simulink model "uz_mpc_cost_and_optim_state_machine"  (R2021a)
settings: Solver=FixedStepAuto  StartTime=0.0  StopTime=10000*t_ADC  RelTol=1e-3
values from neighbouring files (symbols this model uses):
  A = 1.0    (= 1)    [uz_6ph_pu_vsd_voltages_init.m]    (also in uz_mpc_6ph_init.m; uz_mpc_6ph_state_machine_init.m = 0.1)
  f = n_rpm/60.0*p    (= 250)    [uz_6ph_pu_vsd_voltages_init.m]    (also in uz_mpc_6ph_init.m; uz_mpc_6ph_state_machine_init.m = 83.3333333333)
  IB = sqrt(2)*IR    [uz_6ph_pu_vsd_voltages_init.m]    (also in uz_mpc_6ph_init.m; uz_mpc_6ph_state_machine_init.m)
  id_ref = 0.0    (= 0)    [uz_6ph_pu_vsd_voltages_init.m]    (also in uz_mpc_6ph_init.m; uz_mpc_6ph_state_machine_init.m)
  iq_ref = -10.0    (= -10)    [uz_6ph_pu_vsd_voltages_init.m]    (also in uz_mpc_6ph_init.m; uz_mpc_6ph_state_machine_init.m = 5)
  ix_ref = 0.0    (= 0)    [uz_6ph_pu_vsd_voltages_init.m]    (also in uz_mpc_6ph_init.m; uz_mpc_6ph_state_machine_init.m)
  iy_ref = 0.0    (= 0)    [uz_6ph_pu_vsd_voltages_init.m]    (also in uz_mpc_6ph_init.m; uz_mpc_6ph_state_machine_init.m)
  lambda_d = 1.0    (= 1)    [uz_mpc_6ph_state_machine_init.m]
  lambda_q = 1.0    (= 1)    [uz_mpc_6ph_state_machine_init.m]
  lambda_u = 0.0    (= 0)    [uz_mpc_6ph_state_machine_init.m]
  lambda_x = 0.1    [uz_mpc_6ph_state_machine_init.m]
  lambda_y = 0.1    [uz_mpc_6ph_state_machine_init.m]
  Ld_over_LB = Ld/LB    [uz_6ph_pu_vsd_voltages_init.m]    (also in uz_mpc_6ph_init.m; uz_mpc_6ph_state_machine_init.m)
  Lq_over_LB = Lq/LB    [uz_6ph_pu_vsd_voltages_init.m]    (also in uz_mpc_6ph_init.m; uz_mpc_6ph_state_machine_init.m)
  n_rpm = 3000    [uz_6ph_pu_vsd_voltages_init.m]    (also in uz_mpc_6ph_init.m; uz_mpc_6ph_state_machine_init.m = 1000)
  omega_m = n_rpm*pi/30    (= 314.159265359)    [uz_6ph_pu_vsd_voltages_init.m]    (also in uz_mpc_6ph_init.m; uz_mpc_6ph_state_machine_init.m = 104.71975512)
  omegaB = nR*2*pi()/60*p    [uz_6ph_pu_vsd_voltages_init.m]    (also in uz_mpc_6ph_init.m; uz_mpc_6ph_state_machine_init.m)
  p = 5    [uz_6ph_pu_vsd_voltages_init.m]    (also in uz_mpc_6ph_init.m; uz_mpc_6ph_state_machine_init.m)
  psi_pm_over_psiB = psi_pm/psiB    [uz_6ph_pu_vsd_voltages_init.m]    (also in uz_mpc_6ph_init.m; uz_mpc_6ph_state_machine_init.m)
  Rs_over_ZB = Rs/ZB    [uz_6ph_pu_vsd_voltages_init.m]    (also in uz_mpc_6ph_init.m; uz_mpc_6ph_state_machine_init.m)
  t_ADC = 1/f_ADC    (= 1e-05)    [uz_6ph_pu_vsd_voltages_init.m]    (also in uz_mpc_6ph_init.m; uz_mpc_6ph_state_machine_init.m; uz_typeconv_init.m)
  t_clock = 1/f_clock    (= 1e-08)    [uz_6ph_pu_vsd_voltages_init.m]    (also in uz_mpc_6ph_init.m; uz_mpc_6ph_state_machine_init.m; uz_typeconv_init.m)
  Ts_times_ZB_over_Ld = Ts*ZB/Ld    [uz_6ph_pu_vsd_voltages_init.m]    (also in uz_mpc_6ph_init.m; uz_mpc_6ph_state_machine_init.m)
  Ts_times_ZB_over_Lq = Ts*ZB/Lq    [uz_6ph_pu_vsd_voltages_init.m]    (also in uz_mpc_6ph_init.m; uz_mpc_6ph_state_machine_init.m)
  Ts_times_ZB_over_Lx = Ts*ZB/Lx    [uz_6ph_pu_vsd_voltages_init.m]    (also in uz_mpc_6ph_init.m; uz_mpc_6ph_state_machine_init.m)
  Ts_times_ZB_over_Ly = Ts*ZB/Ly    [uz_6ph_pu_vsd_voltages_init.m]    (also in uz_mpc_6ph_init.m; uz_mpc_6ph_state_machine_init.m)
  v_dc = 565.0    (= 565)    [uz_6ph_pu_vsd_voltages_init.m]    (also in uz_mpc_6ph_init.m; uz_mpc_6ph_state_machine_init.m)
  VB = sqrt(2/3)*VR    [uz_6ph_pu_vsd_voltages_init.m]    (also in uz_mpc_6ph_init.m; uz_mpc_6ph_state_machine_init.m)
libraries: nesl_utility x38, fl_lib x30, ee_lib x14, simulink x10, hdlsllib x2
(part 2 of 3)

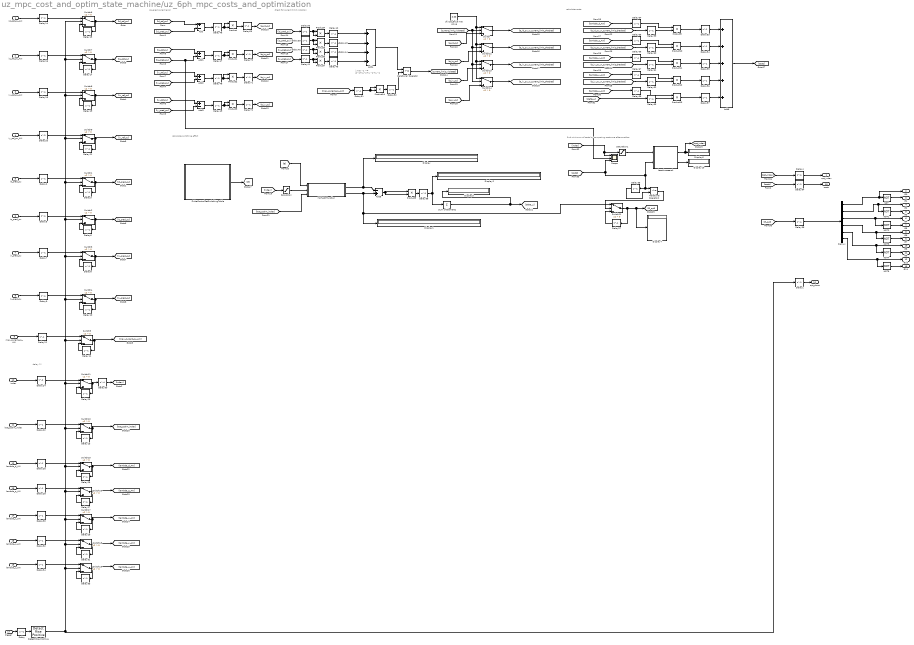
== system uz_mpc_cost_and_optim_state_machine/uz_6ph_mpc_costs_and_optimization ==
  note: delay 2 !
  note: i_max^2 <= id^2+iq^2+ix^2+iy^2
  note: find minimum of costs by comparing costs one after another
  note: calculate costs
  note: calculate switching effort
  note: check for current limit violation
  note: squared current error
  id_ref_pu_AXI : Inport
  iq_ref_pu_AXI : Inport  Port=2
  ix_ref_pu_AXI : Inport  Port=3
  iy_ref_pu_AXI : Inport  Port=4
  id_pred_pu : Inport  Port=5
  iq_pred_pu : Inport  Port=6
  ix_pred_pu : Inport  Port=7
  iy_pred_pu : Inport  Port=8
  max_current_pu_AXI : Inport  Port=9
  index : Inport  Port=10
  last_optim_index : Inport  Port=11
  lambda_d_AXI : Inport  Port=12
  lambda_q_AXI : Inport  Port=13
  lambda_x_AXI : Inport  Port=14
  lambda_y_AXI : Inport  Port=15
  lambda_u_AXI : Inport  Port=16
  trigger : Inport  Port=17
  Add{,1..3} (4 alike) : Sum  Inputs=+-
  Add4 : Sum  Inputs=++++  AccumDataTypeStr=fixdt_type_squared_current_error
  Add5 : Sum  Inputs=-+
  Add6 : Sum  Inputs=+++++  AccumDataTypeStr=fixdt_type_delta_u_costs
  Delay{,1..12,14..21,25..34,36,38..49,51..72,94} (67 alike) : Delay  DelayLength=1
  Delay13 : Delay  DelayLength=1  InitialCondition=1
  Delay22 : Delay  DelayLength=1  InitialCondition=1
  Delay23 : Delay  DelayLength=1  InitialCondition=1
  Delay24 : Delay  InitialCondition=1
  Delay35 : Delay  DelayLength=1  InitialCondition=4.99
  Delay37 : Delay  DelayLength=1  InitialCondition=0
  Delay50 : Delay  DelayLength=4  InitialCondition=1
  Demux : Demux  Outputs=6
  Detect Rise Positive : simulink/Logic and Bit Operations/Detect Rise Positive  vinit=0  OutDataTypeStr=boolean
  Display{,1..3,6..7,10} (7 alike) : Display
  FiniteControlSetSwitchingTable : MATLAB Function  TreatAsAtomicUnit=on
  MATLAB Function : MATLAB Function  TreatAsAtomicUnit=on
  NOT{,1..5} (6 alike) : Logic  Operator=NOT  IconShape=distinctive  AllPortsSameDT=off  OutDataTypeStr=boolean
  Product{,1..7,9..12,14} (13 alike) : Product  OutDataTypeStr=fixdt_type_squared_current_error
  Product13 : Product  OutDataTypeStr=fixdt_type_delta_u_costs
  Product8 : Product  OutDataTypeStr=uint16
  Relational Operator : RelationalOperator  OutDataTypeStr=boolean  RndMeth=Simplest
  Relational Operator1 : RelationalOperator  Operator=<=  OutDataTypeStr=boolean  RndMeth=Simplest
  Saturation : Saturate  UpperLimit=64  LowerLimit=1
  Saturation1 : Saturate  UpperLimit=64  LowerLimit=1
  Scope : Scope  NumInputPorts=3
  Sum of Elements : Sum  Inputs=+  AccumDataTypeStr=uint16
  Switch{,1..19,21} (21 alike) : Switch  Criteria=u2 > Threshold
  iterativesearch : MATLAB Function  TreatAsAtomicUnit=on
  sfix18_En15 max value : Constant  Value=3.99  OutDataTypeStr=fixdt(1,18,15)  SampleTime=-1
  opt_index : Outport  VectorParamsAs1DForOutWhenUnconnected=off
  G0 : Outport  Port=2  VectorParamsAs1DForOutWhenUnconnected=off
  G1 : Outport  Port=3  VectorParamsAs1DForOutWhenUnconnected=off
  G2 : Outport  Port=4  VectorParamsAs1DForOutWhenUnconnected=off
  G3 : Outport  Port=5  VectorParamsAs1DForOutWhenUnconnected=off
  G4 : Outport  Port=6  VectorParamsAs1DForOutWhenUnconnected=off
  G5 : Outport  Port=7  VectorParamsAs1DForOutWhenUnconnected=off
  G6 : Outport  Port=8  VectorParamsAs1DForOutWhenUnconnected=off
  G7 : Outport  Port=9  VectorParamsAs1DForOutWhenUnconnected=off
  G8 : Outport  Port=10  VectorParamsAs1DForOutWhenUnconnected=off
  G9 : Outport  Port=11  VectorParamsAs1DForOutWhenUnconnected=off
  G10 : Outport  Port=12  VectorParamsAs1DForOutWhenUnconnected=off
  G11 : Outport  Port=13  VectorParamsAs1DForOutWhenUnconnected=off
  opt_done : Outport  Port=14  VectorParamsAs1DForOutWhenUnconnected=off
  costs : Outport  Port=15  VectorParamsAs1DForOutWhenUnconnected=off
  wires:
  trigger/1 -> Delay/1
  Delay/1 -> Detect Rise Positive/1
  Delay1/1 -> opt_done/1
  Delay4/1 -> opt_index/1
  Switch9/1 -> [iy_ref_pu], Delay21/1
  Delay17/1 -> Switch7/3
  id_ref_pu_AXI/1 -> Delay14/1
  Delay18/1 -> Switch8/1
  Switch8/1 -> [ix_ref_pu], Delay19/1
  Delay21/1 -> Switch9/3
  Switch7/1 -> [iq_ref_pu], Delay17/1
  iy_ref_pu_AXI/1 -> Delay20/1
  iq_ref_pu_AXI/1 -> Delay16/1
  Delay16/1 -> Switch7/1
  Delay19/1 -> Switch8/3
  Delay20/1 -> Switch9/1
  Delay15/1 -> Switch6/3
  Switch6/1 -> [id_ref_pu], Delay15/1
  ix_ref_pu_AXI/1 -> Delay18/1
  Delay14/1 -> Switch6/1
  Switch1/1 -> [id_pred_pu], Delay3/1
  ix_pred_pu/1 -> Delay7/1
  Delay9/1 -> Switch4/1
  Delay2/1 -> Switch1/1
  Delay8/1 -> Switch3/3
  Delay5/1 -> Switch2/1
  iy_pred_pu/1 -> Delay9/1
  iq_pred_pu/1 -> Delay5/1
  Switch3/1 -> Delay8/1, [ix_pred_pu]
  Delay10/1 -> Switch4/3
  Switch2/1 -> [iq_pred_pu], Delay6/1
  Delay7/1 -> Switch3/1
  Switch4/1 -> [iy_pred_pu], Delay10/1
  Delay6/1 -> Switch2/3
  Delay3/1 -> Switch1/3
  id_pred_pu/1 -> Delay2/1
  max_current_pu_AXI/1 -> Delay12/1
  Delay12/1 -> Switch5/1
  Delay11/1 -> Switch5/3
  Switch5/1 -> [max_current_pu_AXI], Delay11/1
  last_optim_index/1 -> Delay22/1
  Delay22/1 -> Switch10/1
  Delay13/1 -> Switch10/3
  Switch10/1 -> [last_optim_index], Delay13/1
  FiniteControlSetSwitchingTable/1(G) -> [G]
  Delay24/1 -> Switch11/1
  index/1 -> Delay24/1
  Delay23/1 -> Switch11/3
  Switch11/1 -> Delay50/1, Delay23/1
  [e_id_pu] -> Switch/3
  [current_limit_violated] -> Switch13/2, Switch14/2, Switch12/2, Switch/2
  [e_iq_pu] -> Switch12/3
  [e_ix_pu] -> Switch13/3
  sfix18_En15 max value/1 -> Switch/1, Switch14/1, Switch13/1, Switch12/1
  [e_iy_pu] -> Switch14/3
  [G] -> MATLAB Function/1(in)
  Delay26/1 -> Switch15/1
  Delay25/1 -> Switch15/3
  Switch15/1 -> [lambda_d_AXI], Delay25/1
  lambda_d_AXI/1 -> Delay26/1
  lambda_q_AXI/1 -> Delay28/1
  Delay28/1 -> Switch16/1
  Switch16/1 -> [lambda_q_AXI], Delay27/1
  Delay27/1 -> Switch16/3
  lambda_y_AXI/1 -> Delay32/1
  Switch18/1 -> [lambda_y_AXI], Delay31/1
  Delay31/1 -> Switch18/3
  Delay32/1 -> Switch18/1
  lambda_x_AXI/1 -> Delay30/1
  Delay30/1 -> Switch17/1
  Switch17/1 -> [lambda_x_AXI], Delay29/1
  Delay29/1 -> Switch17/3
  Delay33/1 -> Switch19/3
  Switch19/1 -> [lambda_u_AXI], Delay33/1
  lambda_u_AXI/1 -> Delay34/1
  Delay34/1 -> Switch19/1
  [opt_index] -> Delay4/1
  Delay38/1 -> Demux/1
  Add4/1 -> Relational Operator/1
  NOT/1 -> G1/1
  Demux/1 -> G0/1, NOT/1
  NOT5/1 -> G11/1
  NOT4/1 -> G9/1
  NOT3/1 -> G7/1
  NOT2/1 -> G5/1
  NOT1/1 -> G3/1
  Demux/2 -> NOT1/1, G2/1
  Demux/3 -> NOT2/1, G4/1
  Demux/4 -> NOT3/1, G6/1
  Demux/5 -> NOT4/1, G8/1
  Demux/6 -> NOT5/1, G10/1
  Product8/1 -> Delay58/1
  Sum of Elements/1 -> [delta_u], Display3/1
  Add5/1 -> Product8/1, Product8/2
  MATLAB Function/1(G_next) -> Display/1, Add5/1
  Product9/1 -> Delay53/1
  Product10/1 -> Delay54/1
  Product11/1 -> Delay55/1
  Product12/1 -> Delay56/1
  Product13/1 -> Delay57/1
  Add6/1 -> [costs]
  [lambda_d_AXI] -> Delay64/1
  [lambda_q_AXI] -> Delay65/1
  [lambda_x_AXI] -> Delay66/1
  [lambda_y_AXI] -> Delay67/1
  [lambda_u_AXI] -> Delay68/1
  [delta_u] -> Delay63/1
  [e_id_pu_w_current_limit_checked] -> Delay59/1
  [e_iy_pu_w_current_limit_checked] -> Delay62/1
  [e_ix_pu_w_current_limit_checked] -> Delay61/1
  [e_iq_pu_w_current_limit_checked] -> Delay60/1
  [id_ref_pu] -> Add/1
  [id_pred_pu] -> Add/2
  [iq_pred_pu] -> Scope/2, Add1/2
  [iq_ref_pu] -> Add1/1
  [ix_ref_pu] -> Add2/1
  [ix_pred_pu] -> Add2/2
  [iy_ref_pu] -> Add3/1
  [iy_pred_pu] -> Add3/2
  Add3/1 -> Delay49/1
  Add1/1 -> Delay47/1
  Add2/1 -> Delay48/1
  Add/1 -> Delay46/1
  Product3/1 -> Delay72/1
  Product2/1 -> Delay71/1
  Product1/1 -> Delay70/1
  Product/1 -> Delay69/1
  Product4/1 -> Delay42/1
  Product5/1 -> Delay43/1
  Product6/1 -> Delay44/1
  Product7/1 -> Delay45/1
  [id_pred_pu] -> Delay36/1
  [iq_pred_pu] -> Delay39/1
  [ix_pred_pu] -> Delay40/1
  [iy_pred_pu] -> Delay41/1
  Relational Operator/1 -> [current_limit_violated]
  Switch14/1 -> [e_iy_pu_w_current_limit_checked]
  Switch13/1 -> [e_ix_pu_w_current_limit_checked]
  Switch12/1 -> [e_iq_pu_w_current_limit_checked]
  Switch/1 -> [e_id_pu_w_current_limit_checked]
  [max_current_pu_AXI] -> Delay51/1
  Product14/1 -> Delay52/1
  [costs] -> Delay94/1
  Delay94/1 -> costs/1
  Delay37/1 -> Switch21/3
  Switch21/1 -> Display7/1, [G_opt], Delay37/1
  Detect Rise Positive/1 -> Switch4/2, Switch3/2, Switch2/2, Switch1/2, Switch6/2, Switch7/2, Switch8/2, Switch9/2, Switch5/2, Switch11/2, Switch10/2, Switch15/2, Switch16/2, Switch17/2, Switch18/2, Switch19/2, Delay1/1
  MATLAB Function/2(G_prev) -> Add5/2, Display1/1, Switch21/1
  [last_optim_index] -> MATLAB Function/3(last_optim_index)
  [costs] -> Scope/3, Delay35/1, Relational Operator1/1, iterativesearch/2(cost)
  [index] -> Scope/1, Saturation1/1
  [index] -> Saturation/1
  Saturation/1 -> MATLAB Function/2(index)
  Saturation1/1 -> iterativesearch/1(index)
  Delay35/1 -> Relational Operator1/2
  Relational Operator1/1 -> Switch21/2
  [G_opt] -> Delay38/1
  iterativesearch/1(opt_idx) -> [opt_index], Display6/1
  iterativesearch/2(min_costs) -> Display10/1
  Delay36/1 -> Product4/2, Product4/1
  Delay39/1 -> Product5/2, Product5/1
  Delay40/1 -> Product6/2, Product6/1
  Delay41/1 -> Product7/2, Product7/1
  Delay44/1 -> Add4/3
  Delay42/1 -> Add4/1
  Delay45/1 -> Add4/4
  Delay43/1 -> Add4/2
  Delay46/1 -> Product/1, Product/2
  Delay47/1 -> Product1/1, Product1/2
  Delay48/1 -> Product2/1, Product2/2
  Delay49/1 -> Product3/1, Product3/2
  Delay50/1 -> [index]
  Delay51/1 -> Product14/1, Product14/2
  Delay52/1 -> Relational Operator/2
  Delay53/1 -> Add6/1
  Delay54/1 -> Add6/2
  Delay55/1 -> Add6/3
  Delay56/1 -> Add6/4
  Delay57/1 -> Add6/5
  Delay58/1 -> Sum of Elements/1, Display2/1
  Delay59/1 -> Product9/2
  Delay60/1 -> Product10/2
  Delay61/1 -> Product11/2
  Delay62/1 -> Product12/2
  Delay63/1 -> Product13/2
  Delay64/1 -> Product9/1
  Delay65/1 -> Product10/1
  Delay66/1 -> Product11/1
  Delay67/1 -> Product12/1
  Delay68/1 -> Product13/1
  Delay69/1 -> [e_id_pu]
  Delay70/1 -> [e_iq_pu]
  Delay71/1 -> [e_ix_pu]
  Delay72/1 -> [e_iy_pu]

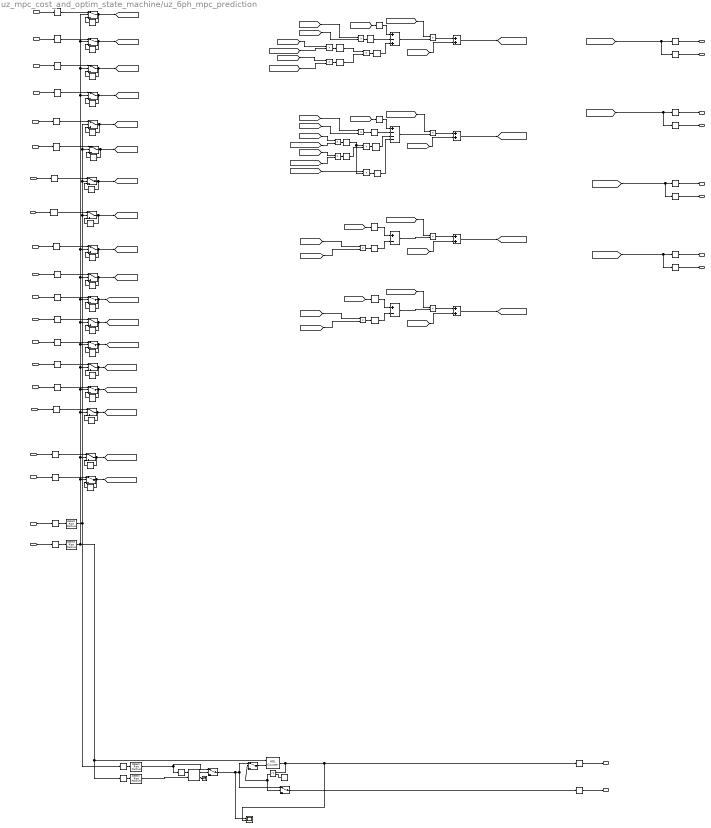
== system uz_mpc_cost_and_optim_state_machine/uz_6ph_mpc_prediction ==
  note: voltages are triggered from voltage calculation ip every iteration
  note: iy_delay_pu = Ts_times_ZB_over_Ly *(vy_pu - Rs_over_ZB * iy_k_pu) + iy_k_pu
  note: ix_delay_pu = Ts_times_ZB_over_Lx *(vx_pu - Rs_over_ZB* ix_k_pu) + ix_k_pu
  note: iq_delay_pu = Ts_times_ZB_over_Lq *(vq_pu - Rs_over_ZB * iq_k_pu - omega_m_pu * polepairs * Ld_over_LB * id_k_pu - omega_m_pu * polepairs * psi_pm_over_psiB) + iq_k_pu
  note: id_delay_pu = Ts_times_ZB_over_Ld *(vd_pu - Rs_over_ZB * id_k_pu + iq_k_pu * Lq_over_LB * omega_m_pu * polepairs) + id_k_pu
  note: mpc state machine
  id_pu : Inport  OutDataTypeStr=fixdt_type_dq_currents
  iq_pu : Inport  Port=2  OutDataTypeStr=fixdt_type_dq_currents
  ix_pu : Inport  Port=3  OutDataTypeStr=fixdt_type_xy_currents
  iy_pu : Inport  Port=4  OutDataTypeStr=fixdt_type_xy_currents
  vd_pu : Inport  Port=5  OutDataTypeStr=fixdt_type_dqxy_voltages
  vq_pu : Inport  Port=6  OutDataTypeStr=fixdt_type_dqxy_voltages
  vx_pu : Inport  Port=7  OutDataTypeStr=fixdt_type_dqxy_voltages
  vy_pu : Inport  Port=8  OutDataTypeStr=fixdt_type_dqxy_voltages
  omega_m_pu : Inport  Port=9  OutDataTypeStr=fixdt_type_speed
  Rs_over_ZB_AXI : Inport  Port=10  OutDataTypeStr=fixdt_type_constants
  Ts_times_ZB_over_Ld_AXI : Inport  Port=11  OutDataTypeStr=fixdt_type_constants
  Ts_times_ZB_over_Lq_AXI : Inport  Port=12  OutDataTypeStr=fixdt_type_constants
  Ts_times_ZB_over_Lx_AXI : Inport  Port=13  OutDataTypeStr=fixdt_type_constants
  Ts_times_ZB_over_Ly_AXI : Inport  Port=14  OutDataTypeStr=fixdt_type_constants
  Ld_over_LB_AXI : Inport  Port=15  OutDataTypeStr=fixdt_type_constants
  Lq_over_LB_AXI : Inport  Port=16  OutDataTypeStr=fixdt_type_constants
  psi_pm_over_psiB_AXI : Inport  Port=17  OutDataTypeStr=fixdt_type_constants
  polepairs_AXI : Inport  Port=18  OutDataTypeStr=fixdt_type_polepairs
  trigger_voltages_done : Inport  Port=19
  adc_trigger : Inport  Port=20
  Add : Sum  Inputs=+-+  AccumDataTypeStr=fixdt(1,27,16)
  Add{1,3,5,7} (4 alike) : Sum  AccumDataTypeStr=fixdt(1,27,24)
  Add2 : Sum  Inputs=+---  AccumDataTypeStr=fixdt(1,27,16)
  Add4 : Sum  Inputs=+-  AccumDataTypeStr=fixdt(1,27,16)
  Add6 : Sum  Inputs=+-  AccumDataTypeStr=fixdt(1,27,16)
  Constant : Constant  Value=63  OutDataTypeStr=uint8  SampleTime=-1
  Delay{,2,4,6,8,11..12,14..17,25,27,29,31,33,35,37,39,43,50,59..60,62..65,71,73} (29 alike) : Delay
  Delay{1,3,5,7,9..10,13,18..24,26,28,30,32,34,36,38,40..42,44..48,53..55,57..58,70,72} (36 alike) : Delay  DelayLength=1
  Delay49 : Delay  DelayLength=1  InitialCondition=0
  Detect Rise Positive{,1..3} (4 alike) : simulink/Logic and Bit Operations/Detect Rise Positive  vinit=0  OutDataTypeStr=boolean
  HDL Counter : hdlsllib/Sources/HDL Counter  CountType=Free running  CountInit=0  CountStep=1  CountMax=64  CountFromType=Initial value  CountFrom=0  CountResetPort=on  CountLoadPort=off  CountEnbPort=on  CountDirPort=off  CountHitOutputPort=off  CountDataType=Unsigned  CountWordLen=8  CountFracLen=0  CountSampTime=1
  Product{,1..2,4..7,9..14} (13 alike) : Product  OutDataTypeStr=fixdt(1,18,15)
  Product3 : Product  OutDataTypeStr=fixdt(1,27,16)
  Product8 : Product  OutDataTypeStr=fixdt(1,27,16)
  Relational Operator : RelationalOperator  Operator=<=  OutDataTypeStr=boolean  RndMeth=Simplest
  Scope : Scope  NumInputPorts=2
  Subsystem : Subsystem
  Switch : Switch  Criteria=u2 > Threshold  OutDataTypeStr=fixdt_type_dq_currents
  Switch1 : Switch  Criteria=u2 > Threshold  OutDataTypeStr=fixdt_type_dq_currents
  Switch{12..19} (8 alike) : Switch  Criteria=u2 > Threshold  OutDataTypeStr=fixdt_type_constants
  Switch2 : Switch  Criteria=u2 > Threshold  OutDataTypeStr=fixdt_type_xy_currents
  Switch21 : Switch  Criteria=u2 > Threshold  OutDataTypeStr=fixdt_type_polepairs
  Switch{28..31} (4 alike) : Switch  Criteria=u2 > Threshold  OutDataTypeStr=fixdt_type_dqxy_voltages
  Switch3 : Switch  Criteria=u2 > Threshold  OutDataTypeStr=fixdt_type_xy_currents
  Switch4 : Switch  Criteria=u2 > Threshold
  Switch5 : Switch  Criteria=u2 > Threshold  OutDataTypeStr=fixdt_type_speed
  Switch6 : Switch  Criteria=u2 > Threshold
  Switch7 : Switch  Criteria=u2 > Threshold
  Terminator1 : Terminator
  id_pred_pu : Outport
  iq_pred_pu : Outport  Port=2
  ix_pred_pu : Outport  Port=3
  iy_pred_pu : Outport  Port=4
  id_pred_pu_AXI : Outport  Port=5
  iq_pred_pu_AXI : Outport  Port=6
  ix_pred_pu_AXI : Outport  Port=7
  iy_pred_pu_AXI : Outport  Port=8
  prediction_done : Outport  Port=9
  index : Outport  Port=10  VectorParamsAs1DForOutWhenUnconnected=off
  wires:
  Add5/1 -> [ix_delay_pu]
  Switch12/1 -> [Rs_over_ZB_AXI], Delay26/1
  Add3/1 -> [iq_delay_pu]
  Add1/1 -> [id_delay_pu]
  Add7/1 -> [iy_delay_pu]
  Delay5/1 -> Switch1/3
  Delay25/1 -> Switch12/1
  Delay59/1 -> Switch28/1
  Delay33/1 -> Switch16/1
  vx_pu/1 -> Delay71/1
  vd_pu/1 -> Delay59/1
  Switch15/1 -> [Ts_times_ZB_over_Lx_AXI], Delay32/1
  Ld_over_LB_AXI/1 -> Delay35/1
  Delay2/1 -> Switch/1
  Switch16/1 -> Delay34/1, [Ts_times_ZB_over_Ly_AXI]
  ix_pu/1 -> Delay6/1
  Delay38/1 -> Switch18/3
  Switch17/1 -> Delay36/1, [Ld_over_LB_AXI]
  Delay9/1 -> Switch3/3
  Switch13/1 -> [Ts_times_ZB_over_Ld_AXI], Delay28/1
  Delay/1 -> Detect Rise Positive/1
  Delay34/1 -> Switch16/3
  Delay44/1 -> Switch21/3
  Delay29/1 -> Switch14/1
  Delay8/1 -> Switch3/1
  Switch29/1 -> [vq_pu], Delay58/1
  Switch3/1 -> [iy_pu], Delay9/1
  polepairs_AXI/1 -> Delay43/1
  Delay72/1 -> Switch31/3
  Delay43/1 -> Switch21/1
  Switch14/1 -> [Ts_times_ZB_over_Lq_AXI], Delay30/1
  Delay28/1 -> Switch13/3
  psi_pm_over_psiB_AXI/1 -> Delay39/1
  Delay58/1 -> Switch29/3
  id_pu/1 -> Delay2/1
  Switch21/1 -> [polepairs_AXI], Delay44/1
  Switch/1 -> [id_pu], Delay3/1
  Delay35/1 -> Switch17/1
  Delay31/1 -> Switch15/1
  Switch28/1 -> [vd_pu], Delay57/1
  Ts_times_ZB_over_Ly_AXI/1 -> Delay33/1
  Delay7/1 -> Switch2/3
  Delay37/1 -> Switch18/1
  Delay4/1 -> Switch1/1
  Switch2/1 -> [ix_pu], Delay7/1
  Delay12/1 -> Switch5/1
  Delay73/1 -> Switch31/1
  Switch31/1 -> Delay72/1, [vy_pu]
  omega_m_pu/1 -> Delay12/1
  Delay6/1 -> Switch2/1
  Delay27/1 -> Switch13/1
  vq_pu/1 -> Delay60/1
  Switch5/1 -> [omega_m_pu], Delay13/1
  Lq_over_LB_AXI/1 -> Delay37/1
  iq_pu/1 -> Delay4/1
  iy_pu/1 -> Delay8/1
  vy_pu/1 -> Delay73/1
  Delay70/1 -> Switch30/3
  Delay60/1 -> Switch29/1
  Switch30/1 -> Delay70/1, [vx_pu]
  Ts_times_ZB_over_Lq_AXI/1 -> Delay29/1
  Delay3/1 -> Switch/3
  Switch18/1 -> Delay38/1, [Lq_over_LB_AXI]
  Delay26/1 -> Switch12/3
  Switch19/1 -> [psi_pm_over_psiB_AXI], Delay40/1
  Ts_times_ZB_over_Lx_AXI/1 -> Delay31/1
  Delay71/1 -> Switch30/1
  Switch1/1 -> [iq_pu], Delay5/1
  Ts_times_ZB_over_Ld_AXI/1 -> Delay27/1
  Delay57/1 -> Switch28/3
  Rs_over_ZB_AXI/1 -> Delay25/1
  Delay39/1 -> Switch19/1
  adc_trigger/1 -> Delay/1
  Delay40/1 -> Switch19/3
  Delay13/1 -> Switch5/3
  Delay32/1 -> Switch15/3
  Delay36/1 -> Switch17/3
  Delay30/1 -> Switch14/3
  Delay11/1 -> prediction_done/1
  [iy_delay_pu] -> Delay17/1, Delay65/1
  [iq_delay_pu] -> Delay15/1, Delay63/1
  [id_delay_pu] -> Delay14/1, Delay62/1
  Delay63/1 -> iq_pred_pu_AXI/1
  Delay65/1 -> iy_pred_pu_AXI/1
  Delay64/1 -> ix_pred_pu_AXI/1
  [ix_delay_pu] -> Delay16/1, Delay64/1
  Delay62/1 -> id_pred_pu_AXI/1
  Delay15/1 -> iq_pred_pu/1
  Delay14/1 -> id_pred_pu/1
  Delay16/1 -> ix_pred_pu/1
  Delay17/1 -> iy_pred_pu/1
  Add/1 -> Product/2
  [Ts_times_ZB_over_Ld_AXI] -> Product/1  "Ts_times_ZB_over_Ld"
  Product/1 -> Add1/1
  [id_pu] -> Add1/2  "id_k_pu"
  [Rs_over_ZB_AXI] -> Product1/1  "Rs_over_ZB"
  [id_pu] -> Product1/2  "id_k_pu"
  [iq_pu] -> Product3/1  "iq_k_pu"
  [Lq_over_LB_AXI] -> Product3/2  "Lq_over_LB"
  [omega_m_pu] -> Product4/1  "omega_m_pu"
  [polepairs_AXI] -> Product4/2  "polepairs"
  [Ts_times_ZB_over_Lq_AXI] -> Product5/1  "Ts_times_ZB_over_Lq"
  [iq_pu] -> Product6/2  "iq_k_pu"
  [Rs_over_ZB_AXI] -> Product6/1  "Rs_over_ZB"
  Add2/1 -> Product5/2
  [omega_m_pu] -> Product9/1  "omega_m_pu"
  [iq_pu] -> Add3/2  "iq_k_pu"
  [id_pu] -> Product8/1  "id_k_pu"
  [Ld_over_LB_AXI] -> Product8/2  "Ld_over_LB"
  [polepairs_AXI] -> Product9/2  "polepairs"
  Product5/1 -> Add3/1
  [psi_pm_over_psiB_AXI] -> Product10/1
  [Ts_times_ZB_over_Lx_AXI] -> Product11/1  "Ts_times_ZB_over_Lx"
  [ix_pu] -> Product12/2  "ix_k_pu"
  [Rs_over_ZB_AXI] -> Product12/1  "Rs_over_ZB"
  Add4/1 -> Product11/2
  [ix_pu] -> Add5/2  "ix_k_pu"
  Product11/1 -> Add5/1
  [Rs_over_ZB_AXI] -> Product14/1  "Rs_over_ZB"
  Add6/1 -> Product13/2
  [iy_pu] -> Add7/2  "iy_k_pu"
  [iy_pu] -> Product14/2  "iy_k_pu"
  [Ts_times_ZB_over_Ly_AXI] -> Product13/1  "Ts_times_ZB_over_Ly"
  Product13/1 -> Add7/1
  Product2/1 -> Delay1/1
  Product1/1 -> Delay10/1
  Delay10/1 -> Add/2
  Delay1/1 -> Add/3
  [vd_pu] -> Delay18/1  "vd_pu"
  Delay18/1 -> Add/1
  [vq_pu] -> Delay19/1  "vq_pu"
  Product7/1 -> Delay21/1
  Product10/1 -> Delay22/1
  Delay22/1 -> Add2/4
  Delay21/1 -> Add2/3
  Delay20/1 -> Add2/2
  Delay19/1 -> Add2/1
  Product6/1 -> Delay20/1
  [vx_pu] -> Delay23/1  "vx_pu"
  Delay23/1 -> Add4/1
  Product12/1 -> Delay24/1
  Delay24/1 -> Add4/2
  [vy_pu] -> Delay41/1  "vy_pu"
  Product14/1 -> Delay42/1
  Delay42/1 -> Add6/2
  Delay41/1 -> Add6/1
  Product4/1 -> Delay45/1
  Product3/1 -> Delay46/1
  Delay46/1 -> Product2/2
  Delay45/1 -> Product2/1
  Product9/1 -> Delay47/1
  Delay47/1 -> Product10/2, Product7/1
  Product8/1 -> Delay48/1
  Delay48/1 -> Product7/2
  Detect Rise Positive1/1 -> Delay53/1, Switch31/2, Switch30/2, Switch29/2, Switch28/2  "delay_comp done"
  trigger_voltages_done/1 -> Delay50/1
  Delay50/1 -> Detect Rise Positive1/1
  Switch7/1 -> Scope/1, Switch6/1, Switch4/1  "trigger_predict"
  Detect Rise Positive/1 -> Switch21/2, Switch19/2, Switch18/2, Switch17/2, Switch16/2, Switch15/2, Switch14/2, Switch13/2, Switch12/2, Switch5/2, Switch3/2, Switch2/2, Switch1/2, Switch/2, Delay54/1, HDL Counter/1
  Detect Rise Positive3/1 -> Subsystem/2(Reset)
  Delay54/1 -> Detect Rise Positive3/1
  Delay55/1 -> Subsystem/1(Set)
  Subsystem/2(!Q) -> Terminator1/1
  Detect Rise Positive2/1 -> Delay55/1, Switch7/1
  Subsystem/1(Q) -> Switch7/2  "Q"
  Delay53/1 -> Detect Rise Positive2/1
  HDL Counter/1 -> Relational Operator/1, Scope/2, Delay49/1
  Delay49/1 -> index/1
  Constant/1 -> Relational Operator/2
  Switch4/1 -> HDL Counter/2
  Relational Operator/1 -> Switch6/2, Switch4/2
  Switch6/1 -> Delay11/1

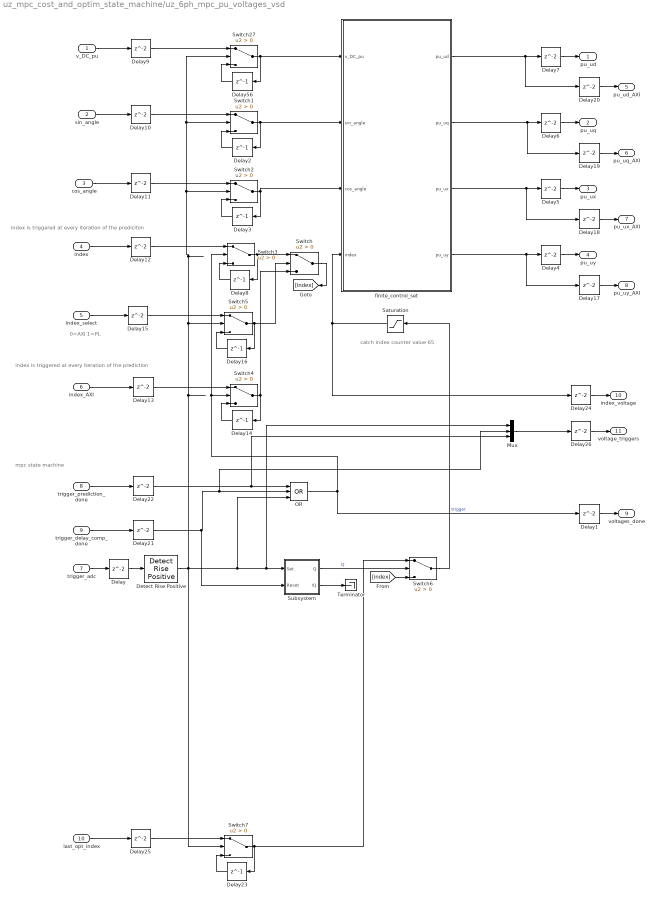
== system uz_mpc_cost_and_optim_state_machine/uz_6ph_mpc_pu_voltages_vsd ==
  note: catch index counter value 65
  note: index is triggered at every iteration of the prediction
  note: index is triggered at every iteration of the prediciton
  note: 0=AXI 1=PL
  note: mpc state machine
  v_DC_pu : Inport  OutDataTypeStr=fixdt_type_constants
  sin_angle : Inport  Port=2  OutDataTypeStr=fixdt_type_sin_cos
  cos_angle : Inport  Port=3  OutDataTypeStr=fixdt_type_sin_cos
  index : Inport  Port=4
  index_select : Inport  Port=5
  index_AXI : Inport  Port=6
  trigger_adc : Inport  Port=7
  trigger_prediction_done : Inport  Port=8
  trigger_delay_comp_done : Inport  Port=9
  last_opt_index : Inport  Port=10
  Delay{,1,4..7,9..11,17..22,24..26} (18 alike) : Delay
  Delay12 : Delay  InitialCondition=0
  Delay13 : Delay  InitialCondition=0
  Delay14 : Delay  DelayLength=1  InitialCondition=0
  Delay15 : Delay  InitialCondition=1
  Delay16 : Delay  DelayLength=1  InitialCondition=1
  Delay2 : Delay  DelayLength=1
  Delay23 : Delay  DelayLength=1  InitialCondition=1
  Delay3 : Delay  DelayLength=1
  Delay56 : Delay  DelayLength=1
  Delay8 : Delay  DelayLength=1  InitialCondition=0
  Detect Rise Positive : simulink/Logic and Bit Operations/Detect Rise Positive  vinit=0  OutDataTypeStr=boolean
  Mux : Mux  Inputs=3
  OR : Logic  Operator=OR  Inputs=3  IconShape=distinctive  AllPortsSameDT=off  OutDataTypeStr=boolean
  Saturation : Saturate  UpperLimit=64  LowerLimit=1
  Subsystem : Subsystem
  Switch : Switch  Criteria=u2 > Threshold
  Switch1 : Switch  Criteria=u2 > Threshold  OutDataTypeStr=fixdt_type_sin_cos
  Switch2 : Switch  Criteria=u2 > Threshold  OutDataTypeStr=fixdt_type_sin_cos
  Switch27 : Switch  Criteria=u2 > Threshold  OutDataTypeStr=fixdt_type_constants
  Switch3 : Switch  Criteria=u2 > Threshold  OutDataTypeStr=fixdt_type_polepairs
  Switch4 : Switch  Criteria=u2 > Threshold  OutDataTypeStr=fixdt_type_polepairs
  Switch5 : Switch  Criteria=u2 > Threshold  OutDataTypeStr=fixdt_type_polepairs
  Switch6 : Switch  Criteria=u2 > Threshold
  Switch7 : Switch  Criteria=u2 > Threshold  OutDataTypeStr=uint32
  Terminator : Terminator
  finite_control_set : MATLAB Function  TreatAsAtomicUnit=on
  pu_ud : Outport
  pu_uq : Outport  Port=2
  pu_ux : Outport  Port=3
  pu_uy : Outport  Port=4
  pu_ud_AXI : Outport  Port=5
  pu_uq_AXI : Outport  Port=6
  pu_ux_AXI : Outport  Port=7
  pu_uy_AXI : Outport  Port=8
  voltages_done : Outport  Port=9
  index_voltage : Outport  Port=10
  voltage_triggers : Outport  Port=11
  wires:
  finite_control_set/1(pu_ud) -> Delay20/1, Delay7/1
  finite_control_set/2(pu_uq) -> Delay19/1, Delay6/1
  finite_control_set/3(pu_ux) -> Delay18/1, Delay5/1
  finite_control_set/4(pu_uy) -> Delay17/1, Delay4/1
  trigger_adc/1 -> Delay/1
  Delay/1 -> Detect Rise Positive/1
  Delay56/1 -> Switch27/3
  v_DC_pu/1 -> Delay9/1
  Switch27/1 -> Delay56/1, finite_control_set/1(v_DC_pu)
  sin_angle/1 -> Delay10/1
  Delay2/1 -> Switch1/3
  Switch1/1 -> finite_control_set/2(sin_angle), Delay2/1
  cos_angle/1 -> Delay11/1
  Delay3/1 -> Switch2/3
  Switch2/1 -> finite_control_set/3(cos_angle), Delay3/1
  Delay4/1 -> pu_uy/1
  Delay5/1 -> pu_ux/1
  Delay6/1 -> pu_uq/1
  Delay7/1 -> pu_ud/1
  Switch3/1 -> Delay8/1, Switch/1
  index/1 -> Delay12/1
  Delay8/1 -> Switch3/3
  Delay9/1 -> Switch27/1
  Delay10/1 -> Switch1/1
  Delay11/1 -> Switch2/1
  Delay12/1 -> Switch3/1
  Delay14/1 -> Switch4/3
  index_AXI/1 -> Delay13/1
  Switch4/1 -> Switch/3, Delay14/1
  Delay13/1 -> Switch4/1
  Delay16/1 -> Switch5/3
  index_select/1 -> Delay15/1
  Switch5/1 -> Switch/2, Delay16/1
  Delay15/1 -> Switch5/1
  Delay17/1 -> pu_uy_AXI/1
  Delay19/1 -> pu_uq_AXI/1
  Delay20/1 -> pu_ud_AXI/1
  Delay18/1 -> pu_ux_AXI/1
  trigger_delay_comp_done/1 -> Delay21/1
  Delay21/1 -> Subsystem/2(Reset), Mux/2, OR/2
  OR/1 -> Switch3/2, Switch4/2, Delay1/1  "trigger"
  Subsystem/2(!Q) -> Terminator/1
  Delay1/1 -> voltages_done/1
  Subsystem/1(Q) -> Switch6/2  "Q"
  Switch/1 -> [index]
  [index] -> Switch6/3
  Switch6/1 -> Saturation/1
  trigger_prediction_done/1 -> Delay22/1
  Saturation/1 -> finite_control_set/4(index), Delay24/1
  Delay24/1 -> index_voltage/1
  last_opt_index/1 -> Delay25/1
  Switch7/1 -> Switch6/1, Delay23/1
  Detect Rise Positive/1 -> Switch7/2, Mux/1, Subsystem/1(Set), OR/3, Switch5/2, Switch2/2, Switch1/2, Switch27/2
  Delay23/1 -> Switch7/3
  Delay25/1 -> Switch7/1
  Delay22/1 -> Mux/3, OR/1
  Delay26/1 -> voltage_triggers/1
  Mux/1 -> Delay26/1

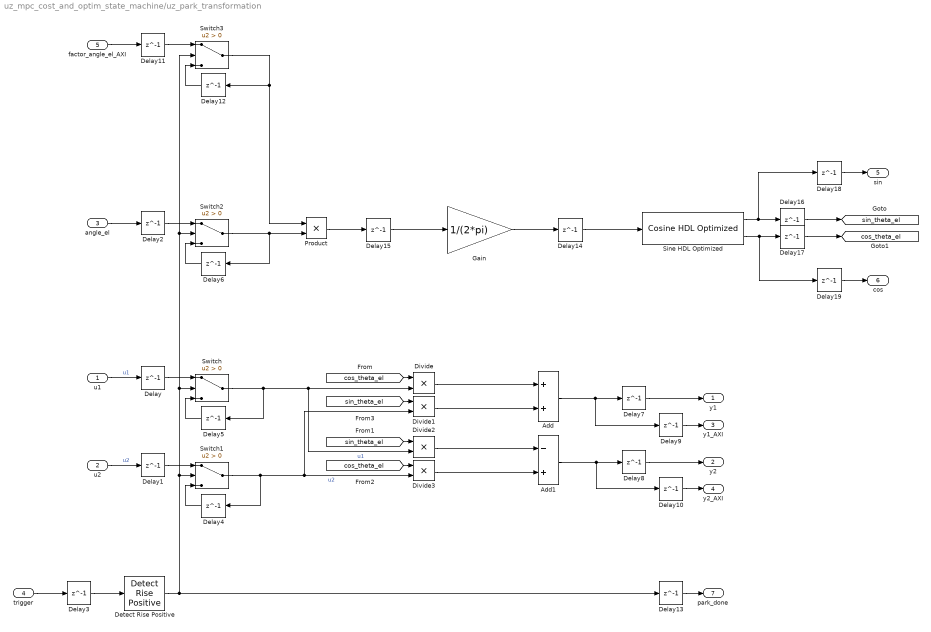
== system uz_mpc_cost_and_optim_state_machine/uz_park_transformation ==
  u1 : Inport
  u2 : Inport  Port=2
  angle_el : Inport  Port=3
  trigger : Inport  Port=4
  factor_angle_el_AXI : Inport  Port=5
  Add : Sum  OutDataTypeStr=fixdt(1,27,16)
  Add1 : Sum  Inputs=-+  OutDataTypeStr=fixdt(1,27,16)
  Delay{,1..19} (20 alike) : Delay  DelayLength=1
  Detect Rise Positive : simulink/Logic and Bit Operations/Detect Rise Positive  vinit=0  OutDataTypeStr=boolean
  Divide{,1..3} (4 alike) : Product  Inputs=**  OutDataTypeStr=fixdt(1,27,16)
  Gain : Gain  Gain=1/(2*pi)  OutDataTypeStr=fixdt(1,18,16)
  Product : Product  OutDataTypeStr=fixdt(1,18,14)
  Sine HDL Optimized : hdlsllib/Lookup Tables/Cosine HDL Optimized  OutputFormula=sin(2*pi*u) and cos(2*pi*u)  NumDataPoints=256  TableDataTypeStr=fixdt(0,17,16)  SimulateLUTROMDelay=off
      settings: SourceProductBaseCode=SL
  Switch{,1..3} (4 alike) : Switch  Criteria=u2 > Threshold
  y1 : Outport  VectorParamsAs1DForOutWhenUnconnected=off
  y2 : Outport  Port=2  VectorParamsAs1DForOutWhenUnconnected=off
  y1_AXI : Outport  Port=3  VectorParamsAs1DForOutWhenUnconnected=off
  y2_AXI : Outport  Port=4  VectorParamsAs1DForOutWhenUnconnected=off
  sin : Outport  Port=5  VectorParamsAs1DForOutWhenUnconnected=off
  cos : Outport  Port=6  VectorParamsAs1DForOutWhenUnconnected=off
  park_done : Outport  Port=7  VectorParamsAs1DForOutWhenUnconnected=off
  tag scope: cos_theta_el=global, sin_theta_el=global
  wires:
  Switch1/1 -> Delay4/1, Divide1/2, Divide3/2  "u2"
  Divide2/1 -> Add1/1
  Divide3/1 -> Add1/2
  [cos_theta_el] -> Divide3/1
  Switch/1 -> Divide2/2, Divide/2, Delay5/1  "u1"
  [sin_theta_el] -> Divide2/1
  Divide1/1 -> Add/2
  [cos_theta_el] -> Divide/1
  [sin_theta_el] -> Divide1/1
  Add/1 -> Delay9/1, Delay7/1
  Add1/1 -> Delay10/1, Delay8/1
  Divide/1 -> Add/1
  angle_el/1 -> Delay2/1
  Sine HDL Optimized/2 -> Delay19/1, Delay17/1
  Sine HDL Optimized/1 -> Delay18/1, Delay16/1
  Gain/1 -> Delay14/1
  u1/1 -> Delay/1  "u1"
  u2/1 -> Delay1/1  "u2"
  Delay/1 -> Switch/1
  Delay1/1 -> Switch1/1
  Delay2/1 -> Switch2/1
  trigger/1 -> Delay3/1
  Delay4/1 -> Switch1/3
  Delay5/1 -> Switch/3
  Delay6/1 -> Switch2/3
  Delay7/1 -> y1/1
  Delay8/1 -> y2/1
  Delay9/1 -> y1_AXI/1
  Delay10/1 -> y2_AXI/1
  Switch2/1 -> Product/2, Delay6/1
  Switch3/1 -> Product/1, Delay12/1
  factor_angle_el_AXI/1 -> Delay11/1
  Detect Rise Positive/1 -> Delay13/1, Switch1/2, Switch/2, Switch3/2, Switch2/2
  Delay12/1 -> Switch3/3
  Delay11/1 -> Switch3/1
  Product/1 -> Delay15/1
  Delay3/1 -> Detect Rise Positive/1
  Delay13/1 -> park_done/1
  Delay15/1 -> Gain/1
  Delay14/1 -> Sine HDL Optimized/1
  Delay16/1 -> [sin_theta_el]
  Delay17/1 -> [cos_theta_el]
  Delay18/1 -> sin/1
  Delay19/1 -> cos/1

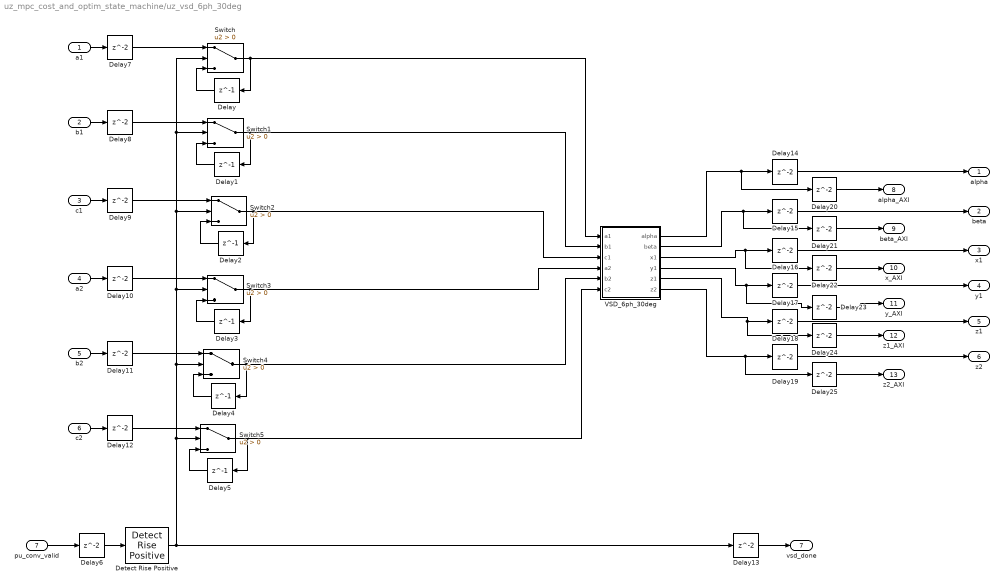
== system uz_mpc_cost_and_optim_state_machine/uz_vsd_6ph_30deg ==
  a1 : Inport
  b1 : Inport  Port=2
  c1 : Inport  Port=3
  a2 : Inport  Port=4
  b2 : Inport  Port=5
  c2 : Inport  Port=6
  pu_conv_valid : Inport  Port=7
  Delay{,1..5} (6 alike) : Delay  DelayLength=1
  Delay{6..25} (20 alike) : Delay
  Detect Rise Positive : simulink/Logic and Bit Operations/Detect Rise Positive  vinit=0  OutDataTypeStr=boolean
  Switch{,1..5} (6 alike) : Switch  Criteria=u2 > Threshold  OutDataTypeStr=fixdt_type_vsd
  VSD_6ph_30deg : MATLAB Function  TreatAsAtomicUnit=on
  alpha : Outport  OutDataTypeStr=fixdt(1,18,11)  VectorParamsAs1DForOutWhenUnconnected=off
  beta : Outport  Port=2  OutDataTypeStr=fixdt(1,18,11)  VectorParamsAs1DForOutWhenUnconnected=off
  x1 : Outport  Port=3  OutDataTypeStr=fixdt(1,18,11)  VectorParamsAs1DForOutWhenUnconnected=off
  y1 : Outport  Port=4  OutDataTypeStr=fixdt(1,18,11)  VectorParamsAs1DForOutWhenUnconnected=off
  z1 : Outport  Port=5  OutDataTypeStr=fixdt(1,18,11)  VectorParamsAs1DForOutWhenUnconnected=off
  z2 : Outport  Port=6  OutDataTypeStr=fixdt(1,18,11)  VectorParamsAs1DForOutWhenUnconnected=off
  vsd_done : Outport  Port=7  VectorParamsAs1DForOutWhenUnconnected=off
  alpha_AXI : Outport  Port=8  OutDataTypeStr=fixdt(1,18,11)  VectorParamsAs1DForOutWhenUnconnected=off
  beta_AXI : Outport  Port=9  OutDataTypeStr=fixdt(1,18,11)  VectorParamsAs1DForOutWhenUnconnected=off
  x_AXI : Outport  Port=10  OutDataTypeStr=fixdt(1,18,11)  VectorParamsAs1DForOutWhenUnconnected=off
  y_AXI : Outport  Port=11  OutDataTypeStr=fixdt(1,18,11)  VectorParamsAs1DForOutWhenUnconnected=off
  z1_AXI : Outport  Port=12  OutDataTypeStr=fixdt(1,18,11)  VectorParamsAs1DForOutWhenUnconnected=off
  z2_AXI : Outport  Port=13  OutDataTypeStr=fixdt(1,18,11)  VectorParamsAs1DForOutWhenUnconnected=off
  wires:
  VSD_6ph_30deg/1(alpha) -> Delay20/1, Delay14/1
  VSD_6ph_30deg/2(beta) -> Delay21/1, Delay15/1
  VSD_6ph_30deg/3(x1) -> Delay22/1, Delay16/1
  VSD_6ph_30deg/4(y1) -> Delay23/1, Delay17/1
  VSD_6ph_30deg/5(z1) -> Delay24/1, Delay18/1
  VSD_6ph_30deg/6(z2) -> Delay25/1, Delay19/1
  pu_conv_valid/1 -> Delay6/1
  Detect Rise Positive/1 -> Switch5/2, Switch4/2, Switch3/2, Switch2/2, Switch1/2, Switch/2, Delay13/1
  Delay/1 -> Switch/3
  Switch/1 -> VSD_6ph_30deg/1(a1), Delay/1
  Delay1/1 -> Switch1/3
  Switch1/1 -> VSD_6ph_30deg/2(b1), Delay1/1
  Delay2/1 -> Switch2/3
  Switch2/1 -> VSD_6ph_30deg/3(c1), Delay2/1
  Delay3/1 -> Switch3/3
  Switch3/1 -> VSD_6ph_30deg/4(a2), Delay3/1
  Delay4/1 -> Switch4/3
  Switch4/1 -> VSD_6ph_30deg/5(b2), Delay4/1
  Delay5/1 -> Switch5/3
  Switch5/1 -> VSD_6ph_30deg/6(c2), Delay5/1
  a1/1 -> Delay7/1
  b1/1 -> Delay8/1
  c1/1 -> Delay9/1
  a2/1 -> Delay10/1
  b2/1 -> Delay11/1
  c2/1 -> Delay12/1
  Delay6/1 -> Detect Rise Positive/1
  Delay7/1 -> Switch/1
  Delay8/1 -> Switch1/1
  Delay9/1 -> Switch2/1
  Delay10/1 -> Switch3/1
  Delay11/1 -> Switch4/1
  Delay12/1 -> Switch5/1
  Delay13/1 -> vsd_done/1
  Delay14/1 -> alpha/1
  Delay15/1 -> beta/1
  Delay16/1 -> x1/1
  Delay17/1 -> y1/1
  Delay18/1 -> z1/1
  Delay19/1 -> z2/1
  Delay20/1 -> alpha_AXI/1
  Delay21/1 -> beta_AXI/1
  Delay22/1 -> x_AXI/1
  Delay23/1 -> y_AXI/1
  Delay24/1 -> z1_AXI/1
  Delay25/1 -> z2_AXI/1

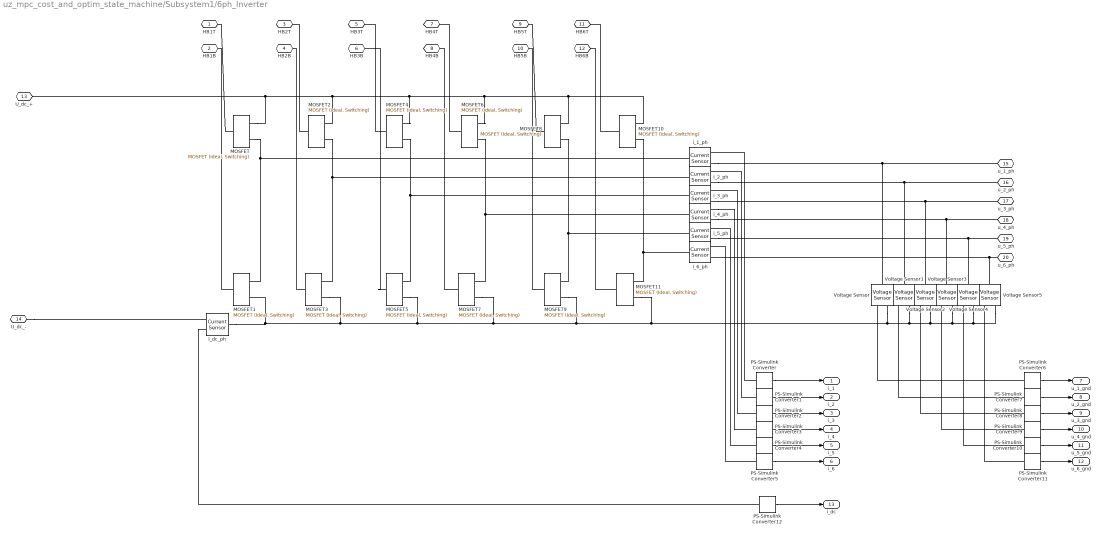
== system uz_mpc_cost_and_optim_state_machine/Subsystem1/6ph_Inverter ==
  MOSFET{,1..11} (12 alike) : ee_lib/Semiconductors & Converters/MOSFET (Ideal, Switching)  Rds=RDSon Ohm  Goff=1e-6 1/Ohm  Vth=0.7 V  diode_param=1  diode_Vf=0.8 V  diode_Ron=0.001 Ohm  diode_Goff=1e-5 1/Ohm  diode_C=5e-8 F  diode_iRM=-235 A  diode_iF=300 A  diode_idot=-50 A/us  diode_trr_param=1  diode_trr_factor=3  diode_trr=15 us  diode_Qrr=1.5e+3 s*uA  thermal_loss_option=ee.enum.converters.thermalLossOption.constantvalues  Von_data=[0, 1.1, 1.3, 1.45, 1.75, 2.25, 2.7; 0, 1, 1.15, 1.35, 1.7, 2.35, 3] V  Eon_data=[0, .29, 1.43, 2.86, 5.71, 13.14, 22.86; 0, .57, 2.63, 5.14, 10.29, 20.57, 30.29] * 1e-3 J  Eoff_data=[0, .21, 1.07, 2.14, 4.29, 9.86, 17.14; 0, .43, 1.97, 3.86, 7.71, 15.43, 22.71] * 1e-3 J  Tj=[298.15, 398.15] K  Iout_data=[0, 10, 50, 100, 200, 400, 600] A  Eon_scalar=22.86e-3 J  Eoff_scalar=17.14e-3 J  Voff=300 V  Iout_scalar=600 A  diodeModelType=ee.enum.converters.diodeModelType.pwl  diode_IfMat=[.07, .12, .19, 1.75, 4.24, 7.32, 11.2; .16, .3, .72, 2.14, 4.02, 6.35, 9.12] A  diode_TjVec=[25, 125] degC  diode_VfVec=[.5, .7, .9, 1.3, 1.7, 2.1, 2.5] V  thermal_network_parameterization=ee.enum.thermalNetworkTopology.external  Rth=[.03, .2] K/W  Rth_Foster=[.03, .2] K/W  thermal_mass_parameterization=ee.enum.thermalNetwork.timeconstant  thermal_mass=[3, 25] J/K  thermal_mass_Foster=[33, 50] J/K  thermal_time_constant=[.1, 5] s  thermal_time_constant_Foster=[1, 10] s  thermal_mass_initial_temperatures=[25, 25] degC  junction_thermal_mass=0.1 J/K  vT_specify=off  vT_priority=None  vT=0 V  vT_nominal_specify=off  vT_nominal_unit=V  vT_nominal_value=1  Qj_specify=off  Qj_priority=None  Qj=0 W  Qj_nominal_specify=off  Qj_nominal_unit=W  Qj_nominal_value=1  junction_temperature_specify=off  junction_temperature_priority=None  junction_temperature=25 degC  junction_temperature_nominal_specify=off  junction_temperature_nominal_unit=degC  junction_temperature_nominal_value=1
  PS-Simulink Converter{,1..5,12} (7 alike) : nesl_utility/PS-Simulink Converter  PhysicalDomain=network_engine_domain  SubClassName=ps_output  LeftPortType=input  RightPortType=output  PseudoPeriodic=off  Frequencies=[]  Unit=A  AffineConversion=off
  PS-Simulink Converter{6..11} (6 alike) : nesl_utility/PS-Simulink Converter  PhysicalDomain=network_engine_domain  SubClassName=ps_output  LeftPortType=input  RightPortType=output  PseudoPeriodic=off  Frequencies=[]  Unit=V  AffineConversion=off
  Voltage Sensor{,1..5} (6 alike) : fl_lib/Electrical/Electrical Sensors/Voltage Sensor
  i_1_ph : fl_lib/Electrical/Electrical Sensors/Current Sensor
  i_2_ph : fl_lib/Electrical/Electrical Sensors/Current Sensor
  i_3_ph : fl_lib/Electrical/Electrical Sensors/Current Sensor
  i_4_ph : fl_lib/Electrical/Electrical Sensors/Current Sensor
  i_5_ph : fl_lib/Electrical/Electrical Sensors/Current Sensor
  i_6_ph : fl_lib/Electrical/Electrical Sensors/Current Sensor
  i_dc_ph : fl_lib/Electrical/Electrical Sensors/Current Sensor
  HB1T : PMIOPort  Side=Left
  HB1B : PMIOPort  Port=2  Side=Left
  HB2T : PMIOPort  Port=3  Side=Left
  HB2B : PMIOPort  Port=4  Side=Left
  HB3T : PMIOPort  Port=5  Side=Left
  HB3B : PMIOPort  Port=6  Side=Left
  HB4T : PMIOPort  Port=7  Side=Left
  HB4B : PMIOPort  Port=8  Side=Left
  HB5T : PMIOPort  Port=9  Side=Left
  HB5B : PMIOPort  Port=10  Side=Left
  HB6T : PMIOPort  Port=11  Side=Left
  HB6B : PMIOPort  Port=12  Side=Left
  U_dc_+ : PMIOPort  Port=13  Side=Left
  U_dc_- : PMIOPort  Port=14  Side=Left
  u_1_ph : PMIOPort  Port=15  Side=Right
  u_2_ph : PMIOPort  Port=16  Side=Right
  u_3_ph : PMIOPort  Port=17  Side=Right
  u_4_ph : PMIOPort  Port=18  Side=Right
  u_5_ph : PMIOPort  Port=19  Side=Right
  u_6_ph : PMIOPort  Port=20  Side=Right
  i_1 : Outport  VectorParamsAs1DForOutWhenUnconnected=off
  i_2 : Outport  Port=2  VectorParamsAs1DForOutWhenUnconnected=off
  i_3 : Outport  Port=3  VectorParamsAs1DForOutWhenUnconnected=off
  i_4 : Outport  Port=4  VectorParamsAs1DForOutWhenUnconnected=off
  i_5 : Outport  Port=5  VectorParamsAs1DForOutWhenUnconnected=off
  i_6 : Outport  Port=6  VectorParamsAs1DForOutWhenUnconnected=off
  u_1_gnd : Outport  Port=7  VectorParamsAs1DForOutWhenUnconnected=off
  u_2_gnd : Outport  Port=8  VectorParamsAs1DForOutWhenUnconnected=off
  u_3_gnd : Outport  Port=9  VectorParamsAs1DForOutWhenUnconnected=off
  u_4_gnd : Outport  Port=10  VectorParamsAs1DForOutWhenUnconnected=off
  u_5_gnd : Outport  Port=11  VectorParamsAs1DForOutWhenUnconnected=off
  u_6_gnd : Outport  Port=12  VectorParamsAs1DForOutWhenUnconnected=off
  i_dc : Outport  Port=13  VectorParamsAs1DForOutWhenUnconnected=off
  wires:
  PS-Simulink Converter/1 -> i_1/1
  PS-Simulink Converter1/1 -> i_2/1
  PS-Simulink Converter2/1 -> i_3/1
  PS-Simulink Converter3/1 -> i_4/1
  PS-Simulink Converter4/1 -> i_5/1
  PS-Simulink Converter5/1 -> i_6/1
  PS-Simulink Converter9/1 -> u_4_gnd/1
  PS-Simulink Converter8/1 -> u_3_gnd/1
  PS-Simulink Converter7/1 -> u_2_gnd/1
  PS-Simulink Converter6/1 -> u_1_gnd/1
  PS-Simulink Converter10/1 -> u_5_gnd/1
  PS-Simulink Converter11/1 -> u_6_gnd/1
  PS-Simulink Converter12/1 -> i_dc/1
  connections:
  MOSFET6/RConn2 -- i_4_ph/LConn1 -- MOSFET7/RConn1
  MOSFET2/RConn2 -- i_2_ph/LConn1 -- MOSFET3/RConn1
  MOSFET4/RConn2 -- i_3_ph/LConn1 -- MOSFET5/RConn1
  MOSFET5/RConn2 -- Voltage Sensor5/RConn2 -- Voltage Sensor4/RConn2 -- Voltage Sensor3/RConn2 -- Voltage Sensor2/RConn2 -- Voltage Sensor1/RConn2 -- Voltage Sensor/RConn2 -- MOSFET11/RConn2 -- MOSFET9/RConn2 -- MOSFET7/RConn2 -- i_dc_ph/LConn1 -- MOSFET1/RConn2 -- MOSFET3/RConn2
  MOSFET/RConn2 -- i_1_ph/LConn1 -- MOSFET1/RConn1
  MOSFET11/LConn1 -- HB6B/RConn1
  MOSFET8/RConn2 -- i_5_ph/LConn1 -- MOSFET9/RConn1
  MOSFET2/LConn1 -- HB2T/RConn1
  MOSFET10/RConn2 -- i_6_ph/LConn1 -- MOSFET11/RConn1
  MOSFET/LConn1 -- HB1T/RConn1
  MOSFET9/LConn1 -- HB5B/RConn1
  MOSFET5/LConn1 -- HB3B/RConn1
  MOSFET1/LConn1 -- HB1B/RConn1
  MOSFET7/LConn1 -- HB4B/RConn1
  MOSFET8/LConn1 -- HB5T/RConn1
  MOSFET4/LConn1 -- HB3T/RConn1
  MOSFET10/LConn1 -- HB6T/RConn1
  MOSFET6/LConn1 -- HB4T/RConn1
  MOSFET3/LConn1 -- HB2B/RConn1
  i_1_ph/RConn2 -- Voltage Sensor/LConn1 -- u_1_ph/RConn1
  i_2_ph/RConn2 -- u_2_ph/RConn1 -- Voltage Sensor1/LConn1
  i_3_ph/RConn2 -- u_3_ph/RConn1 -- Voltage Sensor2/LConn1
  i_4_ph/RConn2 -- Voltage Sensor3/LConn1 -- u_4_ph/RConn1
  i_5_ph/RConn2 -- Voltage Sensor4/LConn1 -- u_5_ph/RConn1
  u_6_ph/RConn1 -- i_6_ph/RConn2 -- Voltage Sensor5/LConn1
  PS-Simulink Converter/LConn1 -- i_1_ph/RConn1
  PS-Simulink Converter1/LConn1 -- i_2_ph/RConn1
  PS-Simulink Converter2/LConn1 -- i_3_ph/RConn1
  i_4_ph/RConn1 -- PS-Simulink Converter3/LConn1
  PS-Simulink Converter4/LConn1 -- i_5_ph/RConn1
  PS-Simulink Converter5/LConn1 -- i_6_ph/RConn1
  PS-Simulink Converter6/LConn1 -- Voltage Sensor/RConn1
  PS-Simulink Converter7/LConn1 -- Voltage Sensor1/RConn1
  PS-Simulink Converter8/LConn1 -- Voltage Sensor2/RConn1
  PS-Simulink Converter9/LConn1 -- Voltage Sensor3/RConn1
  PS-Simulink Converter10/LConn1 -- Voltage Sensor4/RConn1
  PS-Simulink Converter11/LConn1 -- Voltage Sensor5/RConn1
  U_dc_-/RConn1 -- i_dc_ph/RConn2
  PS-Simulink Converter12/LConn1 -- i_dc_ph/RConn1
  MOSFET6/RConn1 -- MOSFET/RConn1 -- U_dc_+/RConn1 -- MOSFET2/RConn1 -- MOSFET4/RConn1 -- MOSFET10/RConn1 -- MOSFET8/RConn1

== system uz_mpc_cost_and_optim_state_machine/Subsystem1/DC_link ==
  Capacitor : fl_lib/Electrical/Electrical Elements/Capacitor  c=C_dc_link uF  r=1e-6 Ohm  g=0 1/Ohm  i_specify=off  i_priority=None  i=0 A  i_nominal_specify=off  i_nominal_unit=A  i_nominal_value=1  v_specify=off  v_priority=None  v=0 V  v_nominal_specify=off  v_nominal_unit=V  v_nominal_value=1  vc_specify=off  vc_priority=High  vc=0 V  vc_nominal_specify=off  vc_nominal_unit=V  vc_nominal_value=1
  PS-Simulink Converter : nesl_utility/PS-Simulink Converter  PhysicalDomain=network_engine_domain  SubClassName=ps_output  LeftPortType=input  RightPortType=output  PseudoPeriodic=off  Frequencies=[]  Unit=1  AffineConversion=off
      settings: SourceProductBaseCode=PW,SS
  Voltage Sensor : fl_lib/Electrical/Electrical Sensors/Voltage Sensor
  U_dc_link+_in : PMIOPort  Side=Left
  U_dc_link-_in : PMIOPort  Port=2  Side=Left
  U_dc_link+_out : PMIOPort  Port=3  Side=Right
  U_dc_link-_out : PMIOPort  Port=4  Side=Right
  u_dc_link_measured : Outport  VectorParamsAs1DForOutWhenUnconnected=off
  wires:
  PS-Simulink Converter/1 -> u_dc_link_measured/1
  connections:
  U_dc_link+_in/RConn1 -- Voltage Sensor/LConn1 -- U_dc_link+_out/RConn1 -- Capacitor/LConn1
  U_dc_link-_in/RConn1 -- Voltage Sensor/RConn2 -- U_dc_link-_out/RConn1 -- Capacitor/RConn1
  Voltage Sensor/RConn1 -- PS-Simulink Converter/LConn1

== system uz_mpc_cost_and_optim_state_machine/Subsystem1/Power_Source ==
  Controlled Voltage Source : fl_lib/Electrical/Electrical Sources/Controlled Voltage Source
  + : PMIOPort  Side=Right
  - : PMIOPort  Port=2  Side=Right
  ref_voltage : PMIOPort  Port=3  Side=Left
  connections:
  Controlled Voltage Source/LConn1 -- +/RConn1
  Controlled Voltage Source/RConn2 -- -/RConn1
  Controlled Voltage Source/RConn1 -- ref_voltage/RConn1

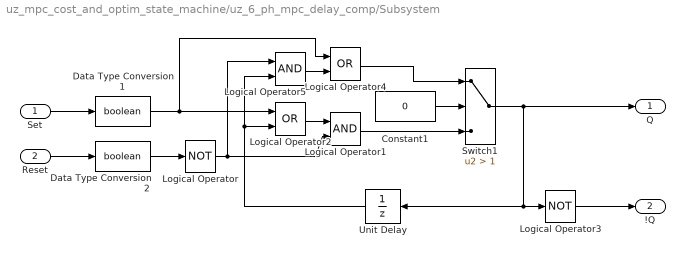
== system uz_mpc_cost_and_optim_state_machine/uz_6_ph_mpc_delay_comp/Subsystem ==
  Set : Inport
  Reset : Inport  Port=2
  Constant1 : Constant  Value=0  OutDataTypeStr=uint32  SampleTime=-1
  Data Type Conversion1 : DataTypeConversion  OutDataTypeStr=boolean
  Data Type Conversion2 : DataTypeConversion  OutDataTypeStr=boolean
  Logical Operator : Logic  Operator=NOT  AllPortsSameDT=off  OutDataTypeStr=boolean
  Logical Operator1 : Logic  AllPortsSameDT=off  OutDataTypeStr=boolean
  Logical Operator2 : Logic  Operator=OR  AllPortsSameDT=off  OutDataTypeStr=boolean
  Logical Operator3 : Logic  Operator=NOT  AllPortsSameDT=off  OutDataTypeStr=boolean
  Logical Operator4 : Logic  Operator=OR  AllPortsSameDT=off  OutDataTypeStr=boolean
  Logical Operator5 : Logic  AllPortsSameDT=off  OutDataTypeStr=boolean
  Switch1 : Switch  Criteria=u2 > Threshold  Threshold=1
  Unit Delay : UnitDelay  InitialCondition=1  SampleTime=t_clock  HasFrameUpgradeWarning=on
  Q : Outport  VectorParamsAs1DForOutWhenUnconnected=off
  !Q : Outport  Port=2  VectorParamsAs1DForOutWhenUnconnected=off
  wires:
  Logical Operator/1 -> Logical Operator1/2, Logical Operator5/1
  Reset/1 -> Data Type Conversion2/1
  Constant1/1 -> Switch1/2
  Logical Operator4/1 -> Switch1/1
  Data Type Conversion1/1 -> Logical Operator2/1, Logical Operator4/1
  Switch1/1 -> Q/1, Unit Delay/1, Logical Operator3/1
  Logical Operator3/1 -> !Q/1
  Set/1 -> Data Type Conversion1/1
  Logical Operator2/1 -> Logical Operator1/1
  Unit Delay/1 -> Logical Operator2/2, Logical Operator5/2
  Logical Operator5/1 -> Logical Operator4/2
  Logical Operator1/1 -> Switch1/3
  Data Type Conversion2/1 -> Logical Operator/1

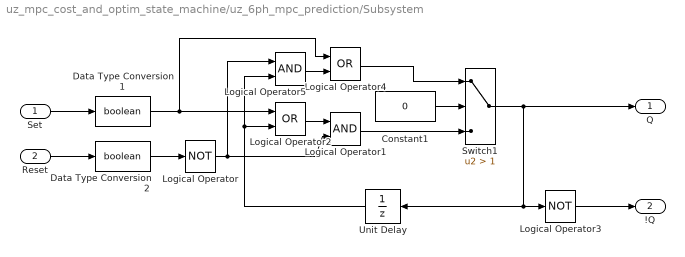
== system uz_mpc_cost_and_optim_state_machine/uz_6ph_mpc_prediction/Subsystem ==
  Set : Inport
  Reset : Inport  Port=2
  Constant1 : Constant  Value=0  OutDataTypeStr=uint32  SampleTime=-1
  Data Type Conversion1 : DataTypeConversion  OutDataTypeStr=boolean
  Data Type Conversion2 : DataTypeConversion  OutDataTypeStr=boolean
  Logical Operator : Logic  Operator=NOT  AllPortsSameDT=off  OutDataTypeStr=boolean
  Logical Operator1 : Logic  AllPortsSameDT=off  OutDataTypeStr=boolean
  Logical Operator2 : Logic  Operator=OR  AllPortsSameDT=off  OutDataTypeStr=boolean
  Logical Operator3 : Logic  Operator=NOT  AllPortsSameDT=off  OutDataTypeStr=boolean
  Logical Operator4 : Logic  Operator=OR  AllPortsSameDT=off  OutDataTypeStr=boolean
  Logical Operator5 : Logic  AllPortsSameDT=off  OutDataTypeStr=boolean
  Switch1 : Switch  Criteria=u2 > Threshold  Threshold=1
  Unit Delay : UnitDelay  SampleTime=t_clock  HasFrameUpgradeWarning=on
  Q : Outport  VectorParamsAs1DForOutWhenUnconnected=off
  !Q : Outport  Port=2  VectorParamsAs1DForOutWhenUnconnected=off
  wires:
  Logical Operator/1 -> Logical Operator1/2, Logical Operator5/1
  Reset/1 -> Data Type Conversion2/1
  Constant1/1 -> Switch1/2
  Logical Operator4/1 -> Switch1/1
  Data Type Conversion1/1 -> Logical Operator2/1, Logical Operator4/1
  Switch1/1 -> Q/1, Unit Delay/1, Logical Operator3/1
  Logical Operator3/1 -> !Q/1
  Set/1 -> Data Type Conversion1/1
  Logical Operator2/1 -> Logical Operator1/1
  Unit Delay/1 -> Logical Operator2/2, Logical Operator5/2
  Logical Operator5/1 -> Logical Operator4/2
  Logical Operator1/1 -> Switch1/3
  Data Type Conversion2/1 -> Logical Operator/1

== system uz_mpc_cost_and_optim_state_machine/uz_6ph_mpc_pu_voltages_vsd/Subsystem ==
  Set : Inport
  Reset : Inport  Port=2
  Constant1 : Constant  Value=0  OutDataTypeStr=uint32  SampleTime=-1
  Data Type Conversion1 : DataTypeConversion  OutDataTypeStr=boolean
  Data Type Conversion2 : DataTypeConversion  OutDataTypeStr=boolean
  Logical Operator : Logic  Operator=NOT  AllPortsSameDT=off  OutDataTypeStr=boolean
  Logical Operator1 : Logic  AllPortsSameDT=off  OutDataTypeStr=boolean
  Logical Operator2 : Logic  Operator=OR  AllPortsSameDT=off  OutDataTypeStr=boolean
  Logical Operator3 : Logic  Operator=NOT  AllPortsSameDT=off  OutDataTypeStr=boolean
  Logical Operator4 : Logic  Operator=OR  AllPortsSameDT=off  OutDataTypeStr=boolean
  Logical Operator5 : Logic  AllPortsSameDT=off  OutDataTypeStr=boolean
  Switch1 : Switch  Criteria=u2 > Threshold  Threshold=1
  Unit Delay : UnitDelay  SampleTime=t_clock  HasFrameUpgradeWarning=on
  Q : Outport  VectorParamsAs1DForOutWhenUnconnected=off
  !Q : Outport  Port=2  VectorParamsAs1DForOutWhenUnconnected=off
  wires:
  Logical Operator/1 -> Logical Operator1/2, Logical Operator5/1
  Reset/1 -> Data Type Conversion2/1
  Constant1/1 -> Switch1/2
  Logical Operator4/1 -> Switch1/1
  Data Type Conversion1/1 -> Logical Operator2/1, Logical Operator4/1
  Switch1/1 -> Q/1, Unit Delay/1, Logical Operator3/1
  Logical Operator3/1 -> !Q/1
  Set/1 -> Data Type Conversion1/1
  Logical Operator2/1 -> Logical Operator1/1
  Unit Delay/1 -> Logical Operator2/2, Logical Operator5/2
  Logical Operator5/1 -> Logical Operator4/2
  Logical Operator1/1 -> Switch1/3
  Data Type Conversion2/1 -> Logical Operator/1
